simulink model "hospital_scenario_before_optimization_simulation"  (R2024b)
settings: Solver=VariableStepAuto  StartTime=0.0  StopTime=100  RelTol=1e-3
undefined symbols (not defined in the file or in its folder): m, n
settings Model: Creator=Alize  LastModifiedBy=Alize

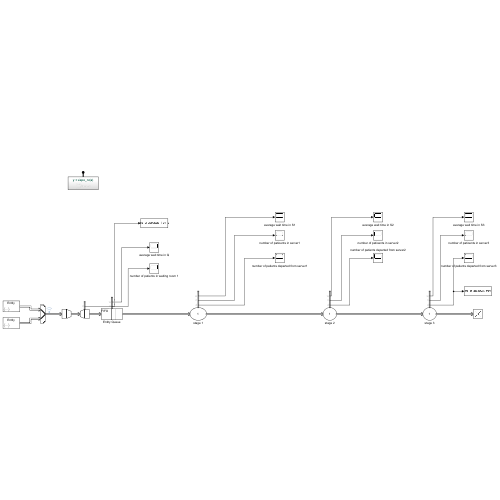
[thumbnail: Simulink's stored preview of the top-level diagram]
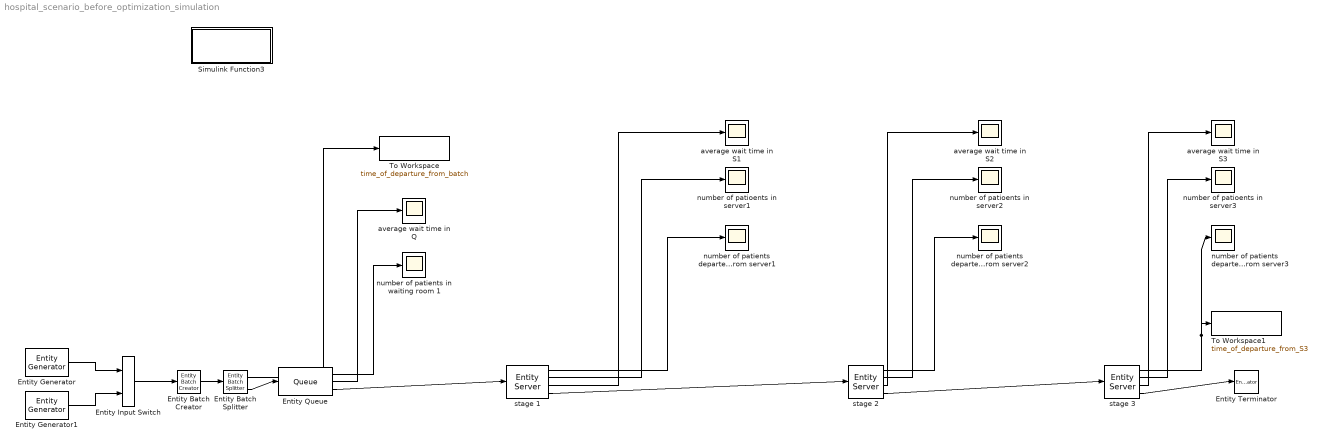
== system hospital_scenario_before_optimization_simulation ==
  Entity Input Switch : EntityInputSwitch  InputPortMessageModes=m,m  OutputPortMessageModes=m
  Entity Batch Creator : EntityBatchCreator  InputPortMessageModes=m  OutputPortMessageModes=m  NumberOfEntitiesInBatch=20
      settings: OutputPortMap=o4
  Entity Batch Splitter : EntityBatchSplitter  InputPortMessageModes=m  OutputPortMessageModes=n,m  NumberOfEntitiesDeparted=on
      settings: OutputPortMap=o1,o4
  Entity Generator : EntityGenerator  OutputPortMessageModes=m  TimeSource=MATLAB action  IntergenerationTimeAction=|  GenerateAction=|  AttributeName=Attribute1|Attribute2  AttributeInitialValue=1|1  EntityType=Structured  EntityTypeName=Entity
      IntergenerationTimeAction=|
      | T = 0;   % fixed intergeneration time
      | N = 10;   % number of entities generated
      | persistent nr;
      | if isempty(nr)
      |   nr = 1;
      | end
      | 
      | if nr <= N
      |   dt = T;
      | else
      |   dt = inf;
      | end
      | nr = nr + 1;
      GenerateAction=|
      | entity.Attribute1 = expo_rv(1);
      | entity.Attribute2 = expo_rv(1/0.5);
  Entity Generator1 : EntityGenerator  OutputPortMessageModes=m  TimeSource=MATLAB action  IntergenerationTimeAction=|  GenerateAction=|  AttributeName=Attribute1|Attribute2  AttributeInitialValue=1|1  EntityType=Structured  EntityTypeName=Entity
      IntergenerationTimeAction=|
      | T = 0;   % fixed intergeneration time
      | N = 10;   % number of entities generated
      | persistent nr;
      | if isempty(nr)
      |   nr = 1;
      | end
      | 
      | if nr <= N
      |   dt = T;
      | else
      |   dt = inf;
      | end
      | nr = nr + 1;
      GenerateAction=|
      | entity.Attribute1 = expo_rv(1/0.5);
      | entity.Attribute2 = expo_rv(1/1.5);
  Entity Queue : Queue  InputPortMessageModes=m  OutputPortMessageModes=n,n,m  Capacity=20  NumberEntitiesInBlock=on  AverageWait=on
      settings: OutputPortMap=o1,o2,o5
  Entity Terminator : EntityTerminator  InputPortMessageModes=m
  Simulink Function3 : Subsystem  TreatAsAtomicUnit=on
  To Workspace : ToWorkspace  VariableName=time_of_departure_from_batch  SaveFormat=Timeseries  SampleTime=-1
  To Workspace1 : ToWorkspace  VariableName=time_of_departure_from_S3  SaveFormat=Timeseries  SampleTime=-1
  average wait time in Q : Scope
  average wait time in S1 : Scope
  average wait time in S2 : Scope
  average wait time in S3 : Scope
  number of patients departed from server1 : Scope
  number of patients departed from server2 : Scope
  number of patients departed from server3 : Scope
  number of patients in waiting room 1 : Scope
  number of patioents in server1 : Scope
  number of patioents in server2 : Scope
  number of patioents in server3 : Scope
  stage 1 : EntityServer  InputPortMessageModes=m  OutputPortMessageModes=n,n,n,m  Capacity=1  ServiceTimeSource=Attribute  ServiceTimeAttributeName=Attribute1  ServiceTimeAction=|  NumberEntitiesDeparted=on  NumberEntitiesInBlock=on  AverageWait=on
      | N = 20;   % number of entities generated
      | persistent nr;
      | if isempty(nr)
      |   nr = 1;
      | end
      | 
      | if nr <= N
      |     for i = 1:20
      |         dt(i) = P1(i);
      |     end
      | else
      |   dt = inf;
      | end
      | nr = nr + 1;
      settings: OutputPortMap=o0,o1,o4,o9
  stage 2 : EntityServer  InputPortMessageModes=m  OutputPortMessageModes=n,n,n,m  Capacity=1  ServiceTimeSource=MATLAB action  ServiceTimeAttributeName=Attribute2  ServiceTimeAction=dt = expo_rv(1/2)  NumberEntitiesDeparted=on  NumberEntitiesInBlock=on  AverageWait=on
      settings: OutputPortMap=o0,o1,o4,o9
  stage 3 : EntityServer  InputPortMessageModes=m  OutputPortMessageModes=n,n,n,m  Capacity=1  ServiceTimeSource=Attribute  ServiceTimeAttributeName=Attribute2  ServiceTimeAction=|  NumberEntitiesDeparted=on  NumberEntitiesInBlock=on  AverageWait=on
      | T = 0;   % fixed intergeneration time
      | N = 20;   % number of entities generated
      | persistent nr;
      | if isempty(nr)
      |   nr = 1;
      | end
      | 
      | if nr <= N
      |   dt = T;
      | else
      |   dt = inf;
      | end
      | nr = nr + 1;
      settings: OutputPortMap=o0,o1,o4,o9
  wires:
  stage 1/3 -> average wait time in S1/1
  Entity Queue/3 -> stage 1/1
  stage 3/3 -> average wait time in S3/1
  Entity Batch Splitter/1 -> To Workspace/1
  stage 3/4 -> Entity Terminator/1
  stage 3/1 -> number of patients departed from server3/1, To Workspace1/1
  stage 2/2 -> number of patioents in server2/1
  stage 1/2 -> number of patioents in server1/1
  stage 2/4 -> stage 3/1
  stage 1/1 -> number of patients departed from server1/1
  Entity Queue/1 -> number of patients in waiting room 1/1
  stage 1/4 -> stage 2/1
  stage 3/2 -> number of patioents in server3/1
  Entity Batch Creator/1 -> Entity Batch Splitter/1
  Entity Queue/2 -> average wait time in Q/1
  Entity Batch Splitter/2 -> Entity Queue/1
  stage 2/1 -> number of patients departed from server2/1
  stage 2/3 -> average wait time in S2/1
  Entity Input Switch/1 -> Entity Batch Creator/1
  Entity Generator/1 -> Entity Input Switch/1
  Entity Generator1/1 -> Entity Input Switch/2

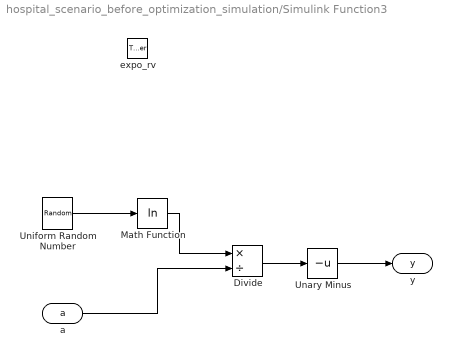
== system hospital_scenario_before_optimization_simulation/Simulink Function3 ==
  expo_rv : TriggerPort  TriggerType=function-call  IsSimulinkFunction=on  FunctionName=expo_rv  FunctionVisibility=scoped  VariantControl=(inherit)
  Divide : Product  Inputs=*/
  Math Function : Math  Operator=log
  Unary Minus : UnaryMinus
  Uniform Random Number : UniformRandomNumber  Minimum=0  VectorParams1D=off
  a : ArgIn  DisableCoverage=on  ArgumentName=a
  y : ArgOut  DisableCoverage=on  ArgumentName=y
  wires:
  a/1 -> Divide/2
  Uniform Random Number/1 -> Math Function/1
  Math Function/1 -> Divide/1
  Divide/1 -> Unary Minus/1
  Unary Minus/1 -> y/1
